simulink model "fir_ma_example_sim"  (R2014a)
settings: Solver=VariableStepDiscrete  StartTime=0.0  StopTime=1  RelTol=1e-3
values from neighbouring files (symbols this model uses):
  dt = 1/Fs    (= 0.0001)    [fiir_matlab_to_C.m]    (also in fir_example.m; fir_ma_example.m = 0.0002; fir_matlab_to_C.m)
  N = max(size(signal))    [fiir_matlab_to_C.m]    (also in fir_ma_example.m = 10; myfir_kaiser_50N_60_600_Hz.m = 50)
undefined symbols (not defined in the file or in its folder): var_n
settings Model: Creator=rodralez  LastModifiedBy=rodralez

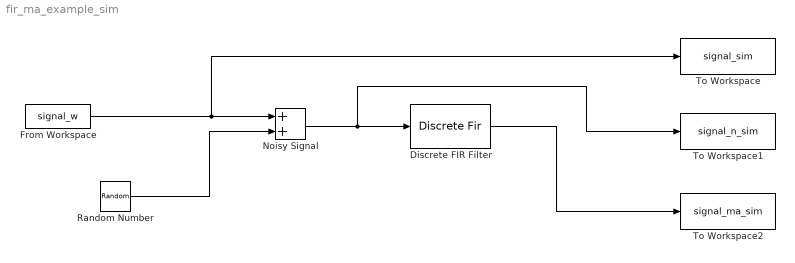
== system fir_ma_example_sim ==
  Discrete FIR Filter : DiscreteFir  Coefficients=ones(1,N)/N  InputProcessing=Columns as channels (frame based)  SampleTime=dt
  From Workspace : FromWorkspace  VariableName=signal_w  SampleTime=dt  Interpolate=off  OutputAfterFinalValue=Setting to zero
  Noisy Signal : Sum  SampleTime=dt
  Random Number : RandomNumber  Variance=var_n  SampleTime=dt
  To Workspace : ToWorkspace  VariableName=signal_sim  SampleTime=-1
      settings: Save2DSignal=2-D array (concatenate along first dimension)
  To Workspace1 : ToWorkspace  VariableName=signal_n_sim  SampleTime=-1
      settings: Save2DSignal=2-D array (concatenate along first dimension)
  To Workspace2 : ToWorkspace  VariableName=signal_ma_sim  SampleTime=-1
      settings: Save2DSignal=2-D array (concatenate along first dimension)
  wires:
  Noisy Signal/1 -> To Workspace1/1, Discrete FIR Filter/1
  From Workspace/1 -> To Workspace/1, Noisy Signal/1
  Random Number/1 -> Noisy Signal/2
  Discrete FIR Filter/1 -> To Workspace2/1
